simulink model "balance_poblacional"  (Simulink 7.5)
settings: Solver=ode1  StartTime=0.0  StopTime=30  FixedStep=0.1  RelTol=1e-3
InitFcn:
  | 'para_inv_prechancado';
  | 'para_inv_prechancado';
  | 'volumen';
settings Model: Creator=vhandaluz  LastModifiedBy=Fer

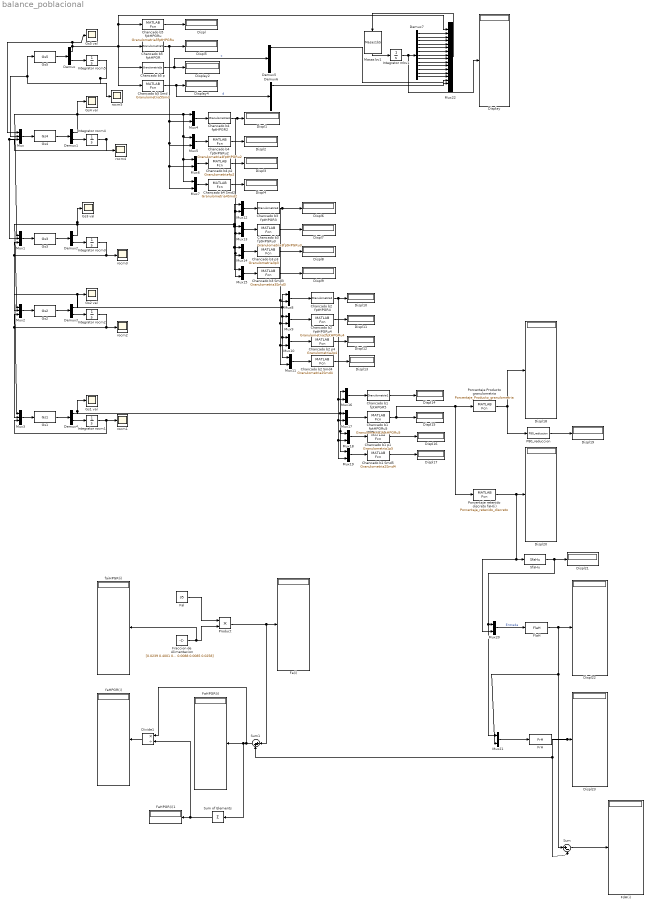
== system balance_poblacional ==
  Chancado b1  fptHPGR5 : MATLABFcn  MATLABFcn=Granulometria1
  Chancado b1  fptHPGRu5 : MATLABFcn  MATLABFcn=Granulometria1fptHPGRu5
  Chancado b1 Smd5 : MATLABFcn  MATLABFcn=Granulometria2Smd4
  Chancado b1 p1 : MATLABFcn  MATLABFcn=Granulometria1p5
  Chancado b2  fptHPGR4 : MATLABFcn  MATLABFcn=Granulometria2
  Chancado b2  fptHPGRu4 : MATLABFcn  MATLABFcn=Granulometria2fptHPGRu4
  Chancado b2 Smd4 : MATLABFcn  MATLABFcn=Granulometria2Smd4
  Chancado b2 p4 : MATLABFcn  MATLABFcn=Granulometria2p4
  Chancado b3  fptHPGR3 : MATLABFcn  MATLABFcn=Granulometria3
  Chancado b3  fptHPGRu3 : MATLABFcn  MATLABFcn=Granulometria3fptHPGRu3
  Chancado b3 Smd3 : MATLABFcn  MATLABFcn=Granulometria3Smd3
  Chancado b3 p3 : MATLABFcn  MATLABFcn=Granulometria3p3
  Chancado b4  fptHPGR2 : MATLABFcn  MATLABFcn=Granulometria4
  Chancado b4  fptHPGRu2 : MATLABFcn  MATLABFcn=Granulometria4fptHPGRu2
  Chancado b4 Smd2 : MATLABFcn  MATLABFcn=Granulometria4Smd2
  Chancado b4 p2 : MATLABFcn  MATLABFcn=Granulometria4p2
  Chancado b5  fptHPGR : MATLABFcn  MATLABFcn=Granulometria5
  Chancado b5 Smd : MATLABFcn  MATLABFcn=Granulometria5Smd
  Chancado b5 fptHPGRu : MATLABFcn  MATLABFcn=Granulometria5fptHPGRu
  Chancado b5 p : MATLABFcn  MATLABFcn=Granulometria5p
  Demux{,1..4} (5 alike) : Demux  Outputs=2
  Demux5 : Demux  Outputs=5
  Demux6 : Demux  Outputs=5
  Demux7 : Demux  Outputs=13
  Displ{,1..23} (24 alike) : Display
  Display : Display
  Display2 : Display
  Display4 : Display
  Divide1 : Product  Inputs=*/  OutDataType=fixdt(1, 16)  OutScaling=2^-10
  Fa(i) : Display
  FaHPGR(i) : Display
  FaHPGR(i)1 : Display
  Fal : Constant  Value=35  OutDataType=fixdt(1, 16)  OutScaling=2^0
  FdH(i) : Display
  FlaH : MATLABFcn  MATLABFcn=FlaH
  FrH : MATLABFcn  MATLABFcn=FrH
  Fraccion de Alimentacion : Constant  Value=[0.0239 0.4001 0.2089 0.1090 0.0549 0.0441 0.0542 0.0374 0.0159 0.0085 0.0088 0.0085 0.0258]  OutDataType=fixdt(1, 16)  OutScaling=2^0
  Gs1 : MATLABFcn  MATLABFcn=Gs1
  Gs1 val : Scope
      settings: SaveName=ScopeData8
  Gs2 : MATLABFcn  MATLABFcn=Gs2
  Gs2 val : Scope
      settings: SaveName=ScopeData6
  Gs3 : MATLABFcn  MATLABFcn=Gs3
  Gs3 val : Scope
      settings: SaveName=ScopeData4
  Gs4 : MATLABFcn  MATLABFcn=Gs4
  Gs4 val : Scope
      settings: SaveName=ScopeData2
  Gs5 : MATLABFcn  MATLABFcn=Gs5
  Gs5 val : Scope
  "Integrator mbv1 " : Integrator  InitialCondition=[4.7411e-6 4.7411e-6 4.7411e-6 4.7411e-6 4.7411e-6 4.7411e-6 4.7411e-6 4.7411e-6 4.7411e-6 4.7411e-6 4.7411e-6 4.7411e-6 4.7411e-6]
  Integrator rocm{1..5} (5 alike) : Integrator  InitialCondition=1.6
  Masas bv1 : MATLABFcn  MATLABFcn=Masas1b5
  Mux{,1..3} (4 alike) : Mux  Inputs=3
  Mux{4..21} (18 alike) : Mux  Inputs=2
  Mux22 : Mux  Inputs=16
  P80_reduccion : MATLABFcn  MATLABFcn=P80_reduccion
  Porcentaje Producto granulometria : MATLABFcn  MATLABFcn=Porcentaje_Producto_granulometria
  Porcentaje retenido discreto faH(i) : MATLABFcn  MATLABFcn=Porcentaje_retenido_discreto
  Product : Product  OutDataType=fixdt(1, 16)  OutScaling=2^0  RndMeth=Zero
  SfaHu : MATLABFcn  MATLABFcn=SfaHu
  Sum : Sum  Inputs=|+-  OutDataType=fixdt(1, 16)  OutScaling=2^0
  Sum of Elements : Sum  Inputs=+  OutDataType=fixdt(1, 16)  OutScaling=2^-10
  Sum1 : Sum  Inputs=|++  OutDataType=fixdt(1, 16)  OutScaling=2^0
  faHPGR(i) : Display
  faiHPGR(i) : Display
  rocm{1..5} (5 alike) : Scope
      rocm1 settings: SaveName=ScopeData9
      rocm2 settings: SaveName=ScopeData7
      rocm3 settings: SaveName=ScopeData5
      rocm4 settings: SaveName=ScopeData3
  wires:
  Integrator rocm5/1 -> rocm5/1, Gs5/1, Mux/2
  Gs5/1 -> Demux/1
  Demux/2 -> Integrator rocm5/1
  Demux/1 -> Mux/1, Gs5 val/1, Chancado b5 p/1, Chancado b5 Smd/1, Chancado b5  fptHPGR/1, Chancado b5 fptHPGRu/1, Mux22/1
  Gs4/1 -> Demux1/1
  Demux1/2 -> Integrator rocm4/1
  Demux1/1 -> Gs4 val/1, Mux1/1, Mux4/1, Mux5/1, Mux6/1, Mux7/1
  Integrator rocm4/1 -> rocm4/1, Mux/3, Mux1/2
  Mux/1 -> Gs4/1
  Gs3/1 -> Demux2/1
  Demux2/2 -> Integrator rocm3/1
  Mux1/1 -> Gs3/1
  Demux2/1 -> Mux2/1, Gs3 val/1, Mux12/1, Mux13/1, Mux14/1, Mux15/1
  Integrator rocm3/1 -> rocm3/1, Mux1/3, Mux2/2
  Mux2/1 -> Gs2/1
  Gs2/1 -> Demux3/1
  Demux3/1 -> Gs2 val/1, Mux3/1, Mux8/1, Mux9/1, Mux10/1, Mux11/1
  Demux3/2 -> Integrator rocm2/1
  Integrator rocm2/1 -> rocm2/1, Mux2/3, Mux3/2
  Mux3/1 -> Gs1/1
  Gs1/1 -> Demux4/1
  Demux4/2 -> Integrator rocm1/1
  Demux4/1 -> Gs1 val/1, Mux16/1, Mux17/1, Mux18/1, Mux19/1
  Integrator rocm1/1 -> Mux3/3, rocm1/1
  Chancado b5 p/1 -> Display2/1, Demux5/1  "c"
  Chancado b5 fptHPGRu/1 -> Displ/1
  Chancado b5 Smd/1 -> Display4/1, Demux6/1  "d"
  Mux4/1 -> Chancado b4  fptHPGR2/1
  Chancado b4  fptHPGR2/1 -> Displ1/1, Mux12/2, Mux13/2, Mux14/2, Mux15/2
  Mux5/1 -> Chancado b4  fptHPGRu2/1
  Mux6/1 -> Chancado b4 p2/1
  Chancado b4 p2/1 -> Displ3/1
  Mux7/1 -> Chancado b4 Smd2/1
  Chancado b4 Smd2/1 -> Displ4/1
  Chancado b5  fptHPGR/1 -> Displ5/1, Mux4/2, Mux5/2, Mux6/2, Mux7/2
  Chancado b4  fptHPGRu2/1 -> Displ2/1
  Mux12/1 -> Chancado b3  fptHPGR3/1
  Mux13/1 -> Chancado b3  fptHPGRu3/1
  Mux14/1 -> Chancado b3 p3/1
  Chancado b3 p3/1 -> Displ8/1
  Mux15/1 -> Chancado b3 Smd3/1
  Chancado b3 Smd3/1 -> Displ9/1
  Chancado b3  fptHPGR3/1 -> Displ6/1, Mux8/2, Mux9/2, Mux10/2, Mux11/2
  Chancado b3  fptHPGRu3/1 -> Displ7/1
  Chancado b2  fptHPGR4/1 -> Displ10/1, Mux16/2, Mux17/2, Mux18/2, Mux19/2
  Mux8/1 -> Chancado b2  fptHPGR4/1
  Chancado b2  fptHPGRu4/1 -> Displ11/1
  Mux9/1 -> Chancado b2  fptHPGRu4/1
  Mux10/1 -> Chancado b2 p4/1
  Chancado b2 p4/1 -> Displ12/1
  Mux11/1 -> Chancado b2 Smd4/1
  Chancado b2 Smd4/1 -> Displ13/1
  Mux16/1 -> Chancado b1  fptHPGR5/1
  Chancado b1  fptHPGR5/1 -> Displ14/1
  Mux17/1 -> Chancado b1  fptHPGRu5/1
  Mux18/1 -> Chancado b1 p1/1
  Chancado b1 p1/1 -> Displ16/1
  Chancado b1 Smd5/1 -> Displ17/1
  Mux19/1 -> Chancado b1 Smd5/1
  Chancado b1  fptHPGRu5/1 -> Displ15/1, Porcentaje Producto granulometria/1, Porcentaje retenido discreto faH(i)/1
  Porcentaje Producto granulometria/1 -> Displ18/1, P80_reduccion/1
  P80_reduccion/1 -> Displ19/1
  Porcentaje retenido discreto faH(i)/1 -> Displ20/1, SfaHu/1, Mux20/2
  SfaHu/1 -> Displ21/1, Mux20/1, Mux21/1
  Mux20/1 -> FlaH/1  "Entrada"
  FlaH/1 -> Displ22/1, Sum/1, Mux21/2
  Mux21/1 -> FrH/1
  FrH/1 -> Displ23/1, Sum/2, Sum1/2
  Sum/1 -> FdH(i)/1
  Fal/1 -> Product/1
  Fraccion de Alimentacion/1 -> Product/2, faiHPGR(i)/1
  Product/1 -> Fa(i)/1, Sum1/1
  Sum1/1 -> FaHPGR(i)/1, Sum of Elements/1, Divide1/1
  Sum of Elements/1 -> FaHPGR(i)1/1, Divide1/2
  Divide1/1 -> faHPGR(i)/1
  "Integrator mbv1 "/1 -> Demux7/1, Display/1
  Mux22/1 -> Masas bv1/1
  Masas bv1/1 -> "Integrator mbv1 "/1
  Demux7/1 -> Mux22/2
  Demux7/2 -> Mux22/3
  Demux7/3 -> Mux22/4
  Demux7/4 -> Mux22/5
  Demux7/5 -> Mux22/6
  Demux7/6 -> Mux22/7
  Demux7/7 -> Mux22/8
  Demux7/8 -> Mux22/9
  Demux7/9 -> Mux22/10
  Demux7/10 -> Mux22/11
  Demux7/11 -> Mux22/12
  Demux7/12 -> Mux22/13
  Demux7/13 -> Mux22/14
  Demux5/1 -> Mux22/15
  Demux6/1 -> Mux22/16
